simulink model "PRegler_Rauschquelle"  (R2025b)
settings: Solver=VariableStepAuto  StartTime=0  StopTime=run_time  MaxStep=1e-5  RelTol=1e-3
values from neighbouring files (symbols this model uses):
  K = 10    [PID_Regler.m]
settings Model: Creator=ruth  LastModifiedBy=ruth

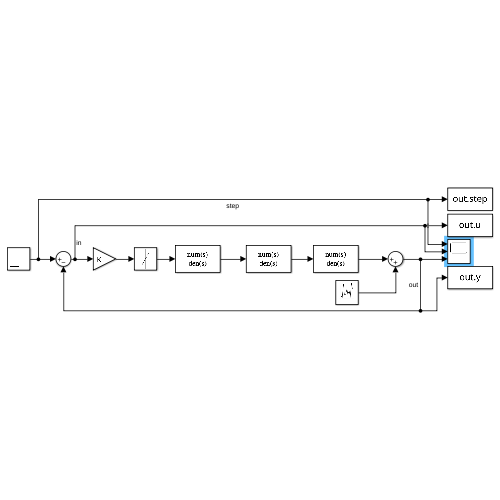
[thumbnail: Simulink's stored preview of the top-level diagram]
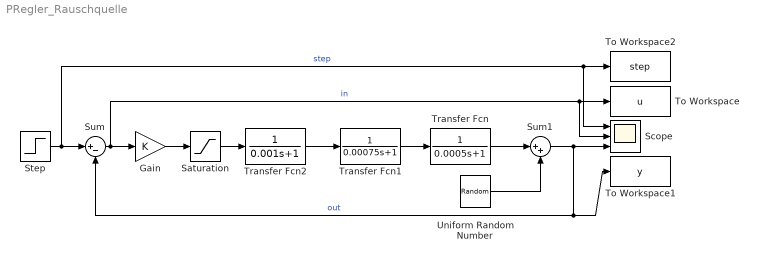
== system PRegler_Rauschquelle ==
  Gain : Gain  Gain=K
  Saturation : Saturate  UpperLimit=12  LowerLimit=-12
  Scope : Scope  NumInputPorts=3
      settings: ActiveDisplayYMinimum=-1.8923972242733083  ActiveDisplayYMaximum=0.05293418809156103
  Step : Step  Time=0  After=0  SampleTime=0
  Sum : Sum  Inputs=|+-
  Sum1 : Sum  Inputs=|++
  To Workspace : ToWorkspace  VariableName=u  SaveFormat=Timeseries  SampleTime=-1
  To Workspace1 : ToWorkspace  VariableName=y  SaveFormat=Timeseries  SampleTime=-1
  To Workspace2 : ToWorkspace  VariableName=step  SaveFormat=Timeseries  SampleTime=-1
  Transfer Fcn : TransferFcn  Denominator=[0.0005 1]
  Transfer Fcn1 : TransferFcn  Denominator=[0.00075 1]
  Transfer Fcn2 : TransferFcn  Denominator=[0.001 1]
  Uniform Random Number : UniformRandomNumber  Minimum=-0.001  Maximum=0.001  SampleTime=0.01
  wires:
  Gain/1 -> Saturation/1
  Saturation/1 -> Transfer Fcn2/1
  Transfer Fcn1/1 -> Transfer Fcn/1
  Transfer Fcn2/1 -> Transfer Fcn1/1
  Sum/1 -> Scope/2, To Workspace/1, Gain/1  "in"
  Step/1 -> Scope/1, To Workspace2/1, Sum/1  "step"
  Uniform Random Number/1 -> Sum1/2
  Transfer Fcn/1 -> Sum1/1
  Sum1/1 -> To Workspace1/1, Sum/2, Scope/3  "out"
